simulink model "SetpointTransitionHandler"  (R2016b)
settings: Solver=FixedStepAuto  StartTime=0.0  StopTime=10.0  RelTol=1e-3  EnableMultiTasking=on
settings Model: Creator=march  LastModifiedBy=snyke7
settings SolverCC: EnableConcurrentExecution=on
settings DataIOCC: SaveFormat=StructureWithTime
settings OptimizationCC: BlockReduction=off  OptimizeBlockIOStorage=off  BufferReuse=off  GlobalBufferReuse=off  ExpressionFolding=off  LocalBlockOutputs=off
settings HardwareCC: ProdBitPerPointer=32  ProdBitPerSizeT=32  ProdBitPerPtrDiffT=32  ProdLargestAtomicFloat=None  ProdWordSize=32  ProdLongLongMode=on  ProdHWDeviceType=Generic->32-bit x86 compatible
settings RTWCC: SystemTargetFile=slrt.tlc  TemplateMakefile=slrt_default_tmf  Description=Simulink Real-Time  RTWCompilerOptimization=on
settings TargetCC: CodeReplacementLibrary=XPC_BLAS  ParMdlRefBuildCompliant=on  ConcurrentExecutionCompliant=on  GeneratePreprocessorConditionals=Use local settings  MatFileLogging=on  MATLABClassNameForMDSCustomization=xpcAperiodicCustomization

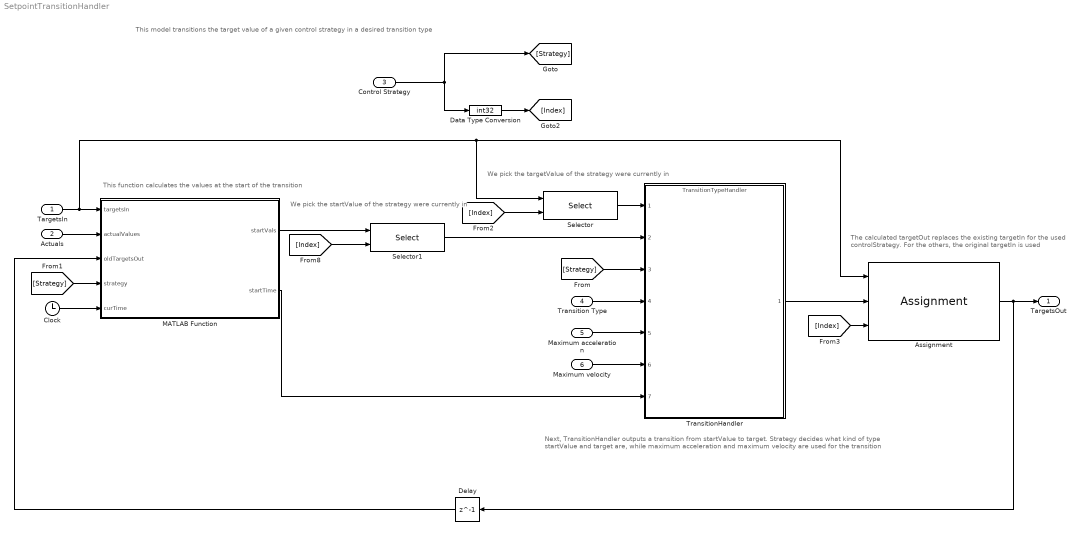
== system SetpointTransitionHandler ==
  note: The calculated targetOut replaces the existing targetIn for the used
      | controlStrategy. For the others, the original targetIn is used
  note: Next, TransitionHandler outputs a transition from startValue to target. Strategy decides what kind of type startValue and target are,
      | while maximum acceleration and maximum velocity are used for the transition
  note: We pick the targetValue of the strategy were currently in
  note: We pick the startValue of the strategy were currently in
  note: This function calculates the values at the start of the transition
  note: This model transitions the target value of a given control strategy in a desired transition type
  TargetsIn : Inport  PortDimensions=[ 3 1 ]
  Actuals : Inport  Port=2  PortDimensions=[ 3 1 ]
  Control Strategy : Inport  Port=3  OutDataTypeStr=Enum: ControlStrategy
  Transition Type : Inport  Port=4
  Maximum acceleration : Inport  Port=5
  Maximum velocity : Inport  Port=6
  Assignment : Assignment  DiagnosticForDimensions=Warning  IndexOptions=Index vector (port)  Indices=1  OutputSizes=1
  Clock : Clock
  Data Type Conversion : DataTypeConversion  OutDataTypeStr=int32
  Delay : Delay  DelayLength=1
  MATLAB Function : MATLAB Function  TreatAsAtomicUnit=on
  Selector : Selector  InputPortWidth=3  IndexOptions=Index vector (port)  Indices=[1 3]  OutputSizes=1
  Selector1 : Selector  InputPortWidth=3  IndexOptions=Index vector (port)  Indices=[1 3]  OutputSizes=1
  TransitionHandler : ModelReference  ModelNameDialog=TransitionTypeHandler  SimulationMode=Normal  ModelReferenceVersion=1.18
  TargetsOut : Outport
  wires:
  Delay/1 -> MATLAB Function/3(oldTargetsOut)
  Actuals/1 -> MATLAB Function/2(actualValues)
  Clock/1 -> MATLAB Function/5(curTime)
  MATLAB Function/2(startTime) -> TransitionHandler/7
  MATLAB Function/1(startVals) -> Selector1/1
  Transition Type/1 -> TransitionHandler/4
  Maximum acceleration/1 -> TransitionHandler/5
  Maximum velocity/1 -> TransitionHandler/6
  TransitionHandler/1 -> Assignment/2
  Assignment/1 -> TargetsOut/1, Delay/1
  Control Strategy/1 -> Data Type Conversion/1, [Strategy]
  [Strategy] -> TransitionHandler/3
  [Strategy] -> MATLAB Function/4(strategy)
  [Index] -> Selector1/2
  [Index] -> Assignment/3
  Data Type Conversion/1 -> [Index]
  Selector1/1 -> TransitionHandler/2
  Selector/1 -> TransitionHandler/1
  TargetsIn/1 -> Selector/1, Assignment/1, MATLAB Function/1(targetsIn)
  [Index] -> Selector/2

== matlab function SetpointTransitionHandler/MATLAB Function ==
  data: targetsIn input; actualValues input; startVals output; oldTargetsOut input; strategy input; curTime input; startTime output
function [startVals, startTime] = getStartValues( targetsIn, actualValues, oldTargetsOut, strategy, curTime)
%% GETSTARTVALUES Outputs startValue of transition from targetsIn to targetsOut
% Outputs the actual value of <target,velocity,position> at the start of
% the transition to targetIn. Also outputs the time this transition was
% initiated

% Initialize persistent variables and constants
persistent oldStart;
persistent prevTime;
persistent oldTargets;
persistent oldStrat;
if isempty(oldStart)
    oldStart = actualValues;
    oldTargets = targetsIn;
    prevTime = curTime;
    oldStrat = strategy;
end
types = [ ControlStrategy.position; ControlStrategy.velocity; ControlStrategy.position ];


% Calculates which targets have reached their desired position. Once this
% has happened, we start updating the startValue again so a next transition
% starts at the right value.
closeEnough = 0.5;
hasReached = abs(targetsIn - oldTargetsOut) < closeEnough;

% The start values should always be the actualValue, unless the given
% control strategy is in transition. If the given control strategy differs
% or the transition is over, use the actualValues:
startVals = or(types ~= strategy, hasReached).*actualValues + ...
    and(types == strategy, not(hasReached)).*oldStart;
% Otherwise (so if the strategy is the control strategy and it is in
% transition, so it h as not reached its target) use the previous
% startValue, which should contain the value when the transition was
% initiated.

% If a target input changed, or the strategy changed, save the currentTime
% into startTime. Otherwise, use the previous startTime
if or(any(oldTargets ~= targetsIn), oldStrat ~= strategy)
    % Note that this currently doesn't support changing a targetValue
    % different from the current strategy. However, in our current setup
    % this always happens both
    startTime = curTime;
else
    startTime = prevTime;
end

% Save the used values for use in the next iteration
oldStart = startVals;
oldTargets = targetsIn;
oldStrat = strategy;
prevTime = startTime;
end
